simulink model "LQR_Test"  (R2013a)
settings: Solver=ode45  StartTime=0.0  StopTime=50  FixedStep=0.01  RelTol=1e-3
values from neighbouring files (symbols this model uses):
  A11 = PA1*A1*PA1^-1    [LQR_Calc.m]    (also in LQR_Calc1.m; LQR_Calc2.m; LQR_Calc2_190m.m; LQR_Calc_Lidawei.m = [-0.0075	0.7497	0	-9.806	0.0001	0	0	0.0328)
  B12 = B11*PU^-1    [LQR_Calc.m]    (also in LQR_Calc1.m; LQR_Calc2.m; LQR_Calc2_190m.m; LQR_Calc_Lidawei.m = [0	0)
  C0 = eye(8)    [LQR_Calc.m]    (also in LQR_Calc1.m; LQR_Calc2.m; LQR_Calc2_190m.m; LQR_Calc_Lidawei.m)
  C11 = [1	0	0	0	0	0	0	0 ... (first row only)    [LQR_Calc.m]    (also in LQR_Calc1.m; LQR_Calc2.m; LQR_Calc2_190m.m = [0	0	0	1	0	0	0	0; LQR_Calc_Lidawei.m = [0	0	0	0	1	0	0	0)
  D = [0 ... (first row only)    [F16AltitudeAutopilotDesign.m]    (also in F16AltitudeAutopilotDesign2.m = [0	0; F16AltitudeAutopilotDesign2_addVilocity.m = [0	0; F16AltitudeAutopilotDesign2_vhold.m = [0	0; F16AltitudeAutopilotDesign_test.m = [0	0)
  KI = k(:,9:10)*2    [LQR_Calc.m]    (also in LQR_Calc1.m = k(:,9:10); LQR_Calc_Lidawei.m = [0.0574,-0.0032; LidaweiPaperTest.m = [0.0574,-0.0032; LidaweiPaperTest2.m = [0.0574,-0.0032)
  KP = k(:,1:8)    [LQR_Calc.m]    (also in LQR_Calc1.m; LQR_Calc_Lidawei.m = [-0.01,-18.7722,1.8698,23.5796,0.1322,-0.0117,3.5775,-0.0001; LidaweiPaperTest.m = [-0.01,-18.7722,1.8698,23.5796,0.1322,-0.0117,3.5775,-0.0001; LidaweiPaperTest2.m = [-0.01,-18.7722,1.8698,23.5796,0.1322,-0.0117,3.5775,-0.0001)
  x0 = [0 0 0 0 0 0 0 0 ]'    [LQR_Calc.m]    (also in LQR_Calc1.m; LQR_Calc_Lidawei.m)
settings Model: Creator=Dai  LastModifiedBy=Dai

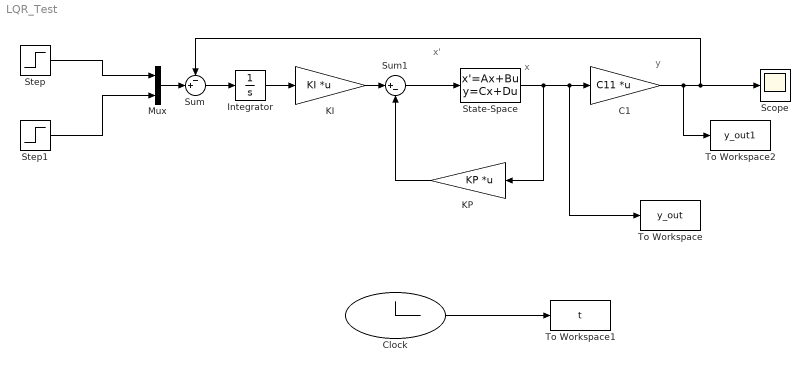
== system LQR_Test ==
  note: y
  note: x'
  note: x
  C1 : Gain  Gain=C11  Multiplication=Matrix(K*u) (u vector)
  Clock : Clock
  Integrator : Integrator
  KI : Gain  Gain=KI  Multiplication=Matrix(K*u) (u vector)
  KP : Gain  Gain=KP  Multiplication=Matrix(K*u) (u vector)
  Mux : Mux  Inputs=2
  Scope : Scope
  State-Space : StateSpace  A=A11  B=B12  C=C0  D=D  X0=x0
  Step : Step  Time=20  After=0  SampleTime=0.001
  Step1 : Step  Time=20  After=0.1  SampleTime=0.001
  Sum : Sum  Inputs=-+|
  Sum1 : Sum  Inputs=|+-
  To Workspace : ToWorkspace  VariableName=y_out  SampleTime=-1
  To Workspace1 : ToWorkspace  VariableName=t  SampleTime=-1
  To Workspace2 : ToWorkspace  VariableName=y_out1  SampleTime=-1
  wires:
  State-Space/1 -> KP/1, To Workspace/1, C1/1
  C1/1 -> To Workspace2/1, Scope/1, Sum/1
  Mux/1 -> Sum/2
  KI/1 -> Sum1/1
  KP/1 -> Sum1/2
  Clock/1 -> To Workspace1/1
  Sum1/1 -> State-Space/1
  Sum/1 -> Integrator/1
  Integrator/1 -> KI/1
  Step/1 -> Mux/1
  Step1/1 -> Mux/2
